simulink model "DLCI"  (R2024a)
settings: Solver=FixedStepDiscrete  StartTime=0.0  StopTime=10.0  FixedStep=.01  RelTol=1e-3
settings Model: Creator=User  LastModifiedBy=User
settings OptimizationCC: DefaultParameterBehavior=Inlined  EnhancedBackFolding=on  PassReuseOutputArgsAs=Individual arguments  ZeroExternalMemoryAtStartup=off  ZeroInternalMemoryAtStartup=off  OptimizeBlockOrder=speed  DifferentSizesBufferReuse=on  OptimizationCustomize=off  EfficientTunableParamExpr=on
settings DebuggingCC: ParameterTunabilityLossMsg=error
settings SFSimCC: MATLABDynamicMemAlloc=off
settings RTWCC: Description=Embedded Coder  SystemTargetFile=ert.tlc  GenCodeOnly=on  TemplateMakefile=ert_default_tmf  GenerateReport=on  LaunchReport=on  GenerateCodeMetricsReport=on
settings CodeAppCC: ForceParamTrailComments=on  IgnoreCustomStorageClasses=off  OperatorAnnotations=on  SimulinkDataObjDesc=on  SFDataObjDesc=on  InsertBlockDesc=on
settings ERTTargetCC: TargetLangStandard=C99 (ISO)  GenerateSampleERTMain=on  InlinedParameterPlacement=NonHierarchical  ERTCustomFileTemplate=example_file_process.tlc

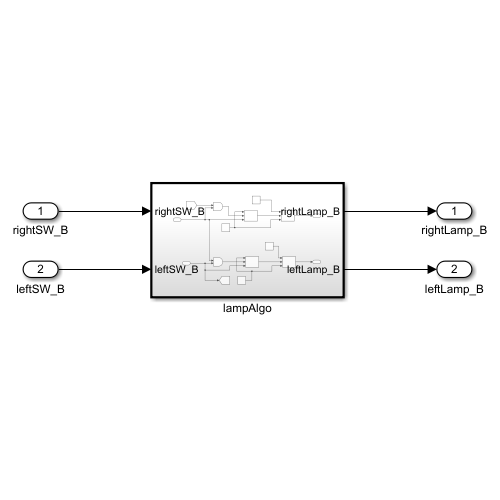
[thumbnail: Simulink's stored preview of the top-level diagram]
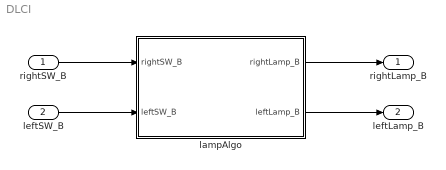
== system DLCI ==
  rightSW_B : Inport  OutDataTypeStr=boolean
  leftSW_B : Inport  Port=2  OutDataTypeStr=boolean
  lampAlgo : Subsystem  TreatAsAtomicUnit=on
      settings: RTWFcnNameOpts=Use subsystem name  RTWFileNameOpts=Use subsystem name
  rightLamp_B : Outport  OutDataTypeStr=boolean
  leftLamp_B : Outport  Port=2  OutDataTypeStr=boolean
  wires:
  rightSW_B/1 -> lampAlgo/1(rightSW_B)
  leftSW_B/1 -> lampAlgo/2(leftSW_B)
  lampAlgo/1(rightLamp_B) -> rightLamp_B/1
  lampAlgo/2(leftLamp_B) -> leftLamp_B/1

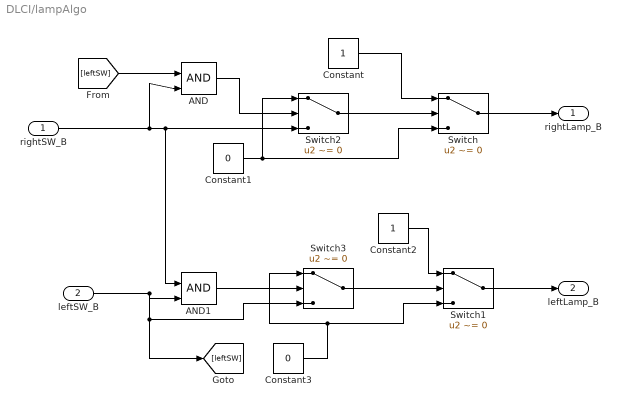
== system DLCI/lampAlgo ==
  rightSW_B : Inport  OutDataTypeStr=boolean
  leftSW_B : Inport  Port=2  OutDataTypeStr=boolean
  AND : Logic  IconShape=distinctive  AllPortsSameDT=off  OutDataTypeStr=boolean
  AND1 : Logic  IconShape=distinctive  AllPortsSameDT=off  OutDataTypeStr=boolean
  Constant : Constant  OutDataTypeStr=boolean
  Constant1 : Constant  Value=0  OutDataTypeStr=boolean
  Constant2 : Constant  OutDataTypeStr=boolean
  Constant3 : Constant  Value=0  OutDataTypeStr=boolean
  Switch{,1..3} (4 alike) : Switch  Criteria=u2 ~= 0  SaturateOnIntegerOverflow=off  InputSameDT=off
  rightLamp_B : Outport  OutDataTypeStr=boolean
  leftLamp_B : Outport  Port=2  OutDataTypeStr=boolean
  wires:
  Switch/1 -> rightLamp_B/1
  Constant/1 -> Switch/1
  Constant1/1 -> Switch2/1, Switch/3
  Switch2/1 -> Switch/2
  AND/1 -> Switch2/2
  [leftSW] -> AND/1
  Switch3/1 -> Switch1/2
  Constant2/1 -> Switch1/1
  Switch1/1 -> leftLamp_B/1
  rightSW_B/1 -> AND1/1, Switch2/3, AND/2
  leftSW_B/1 -> AND1/2, Switch3/3, [leftSW]
  AND1/1 -> Switch3/2
  Constant3/1 -> Switch3/1, Switch1/3
